simulink model "dspintrpfp"  (Simulink 6.0)
settings: Solver=FixedStepDiscrete  SolverMode=SingleTasking  StartTime=0.0  StopTime=50.0  RelTol=1e-3  AbsTol=1e-6
undefined symbols (not defined in the file or in its folder): intfilt
libraries: dspmlti3 x2, dspsigops x1, dspsrcs4 x1
Description:
  | Interpolation based on multirate filtering.
settings Model: CovMetricSettings=d  Creator=don  LastModifiedBy=sconahan  ExtModeTrigMode=oneshot  ExtModeArmWhenConnect=off
settings DataIOCC: LimitDataPoints=off  SaveOutput=off  SaveTime=off  SignalLoggingName=sigsOut
settings OptimizationCC: BlockReduction=off  BooleanDataType=off  MultiInstanced=off  RollThreshold=2
settings FormatCC: IgnoreBidirectionalLines=off
settings DebuggingCC: SingleTaskRateTransMsg=error  IntegerOverflowMsg=none  ParameterPrecisionLossMsg=none
settings HardwareCC: TargetUnknown=on
settings CodeAppCC: FileBanners=off  CustomSymbols=off
settings GRTTargetCC: TargetFcnLib=iso_c_tmw.mat  IsERTTarget=off

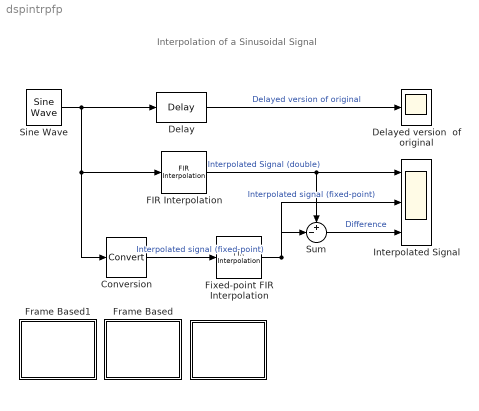
== system dspintrpfp ==
  note: Interpolation of a Sinusoidal Signal
  " " : Subsystem
      mask Type: Interpolation filter info block
      mask Display: disp('Info')
  Conversion : DataTypeConversion  OutDataTypeMode=Specify via dialog  OutScaling=2^-14  RndMeth=Nearest  SaturateOnIntegerOverflow=on
  Delay : dspsigops/Delay  dly_unit=Samples  delay=9  ic_detail=on  dif_ic_for_ch=off  dif_ic_for_dly=off  ic=0  reset_popup=None
  Delayed version  of original : Scope
      settings: TickLabels=on  YMin=-1.2  YMax=1.2  DataFormat=Array
  FIR Interpolation : dspmlti3/FIR Interpolation  h=intfilt(9, 9, .5)  L=9  framing=Maintain input frame size  outputBufInitCond=0  roundingMode=Floor  overflowMode=off
  Fixed-point FIR Interpolation : dspmlti3/FIR Interpolation  h=intfilt(9, 9, .5)  L=9  framing=Maintain input frame size  outputBufInitCond=0  roundingMode=Nearest  overflowMode=off
  Frame Based : Subsystem
      settings: OpenFcn=dspintrpf;
      mask Display: disp('Frame-based\nVersion')
  Frame Based1 : Subsystem
      settings: OpenFcn=dspintrp
      mask Display: disp('Sample-based\nVersion')
  Interpolated Signal : Scope  NumInputPorts=3
      settings: TickLabels=on  TimeRange=50  YMin=-1~-1~-0.0005  YMax=1~1~0.0005  SaveName=ScopeData2  DataFormat=Array
  Sine Wave : dspsrcs4/Sine Wave  Amplitude=1  Frequency=0.2  Phase=0.7  SampleMode=Discrete  OutComplex=Real  CompMethod=Table lookup  TableSize=Speed  SampleTime=1  SamplesPerFrame=1  dataType=double  wordLen=16  udDataType=sfix(16)  fracBitsMode=Best precision  numFracBits=15  ResetState=Restart at time zero
  Sum : Sum  Inputs=+-|  RndMeth=Nearest  SaturateOnIntegerOverflow=on
  wires:
  Sine Wave/1 -> FIR Interpolation/1, Conversion/1, Delay/1
  Delay/1 -> Delayed version  of original/1  "Delayed version of original"
  FIR Interpolation/1 -> Interpolated Signal/1, Sum/1  "Interpolated Signal (double)"
  Fixed-point FIR Interpolation/1 -> Interpolated Signal/2, Sum/2  "Interpolated signal (fixed-point)"
  Sum/1 -> Interpolated Signal/3  "Difference"
  Conversion/1 -> Fixed-point FIR Interpolation/1  "Interpolated signal (fixed-point)"

== system dspintrpfp/  ==
  note: Interpolation of a Sinusoidal Signal
      |
      | The fixed-point FIR Interpolator is based on a polyphase implementation
      | of a FIR interpolation filter (with a factor of 9 upsampling rate).  Notice that each
      |  polyphase FIR filter in the sub-system 'Fixed-point FIR implementation' is a
      |  down-sampled version (by a factor of 9) of the input filter.
      | Effects of  the fixed-point  implementation may be explored by modifying the parameters:
      | Fixed-point word length and fixed-point fractional bits.

== system dspintrpfp/Frame Based ==

== system dspintrpfp/Frame Based1 ==
